simulink model "HSat_orbit"  (R2023a)
settings: Solver=FixedStepAuto  StartTime=0  StopTime=86400*900  MaxStep=3600  RelTol=1e-3  EnableMultiTasking=on
values from neighbouring files (symbols this model uses):
  ext_ENV_G = 6.674e-11    [HSat_op_setup.m]    (also in HSat_op_setup_merged_maria.m)
  ext_ENV_muEarth = 3.986005e14    (= 398600500000000)    [GEO_insertion_setup.m]    (also in HSat_op_setup.m; HSat_op_setup_merged_maria.m; init_orbit_analysis_with_drag_loss.m)
  ext_ENV_Re = 6.37813700*10^6    (= 6378137)    [HSat_op_setup.m]    (also in HSat_op_setup_merged_maria.m)
  ext_EOR_atmosphere_end = 1000e3    (= 1000000)    [HSat_op_setup.m]    (also in HSat_op_setup_merged_maria.m)
  ext_EOR_perigeeraise_end = 600e3    (= 600000)    [HSat_op_setup.m]    (also in HSat_op_setup_merged_maria.m)
  ext_Main_initDate_IC_T = sim_start    [HSat_op_setup.m]    (also in HSat_op_setup_merged_maria.m)
  ext_SC_activecorr_COE_ECI = [1, 1, 1, 0, 0, 0, 0, 0 ]    [HSat_op_setup.m]    (also in HSat_op_setup_merged_maria.m)
  ext_SC_balanced_COE_ECI = [ .500    0.70    1.100 1 1]    [HSat_op_setup.m]    (also in HSat_op_setup_merged_maria.m = [ 0.10 2.10 1.40    1.0000    1.0000]; launch_settings.m)
  ext_SC_cutofferror_COE_ECI = [150e3, .01, 0.1*pi/180, .1*pi/180,.1*pi/180, 0, 0, 0]    [HSat_op_setup.m]    (also in HSat_op_setup_merged_maria.m)
  ext_SC_init_COE_ECI = [a0,ecc0,i0,an0,ap0,tran0,eccan0,ma0]    [HSat_op_setup.m]    (also in HSat_op_setup_merged_maria.m)
  ext_SC_target_COE_ECI = [a1,ecc1,i1,an1,ap1,tran1,eccan1,ma1]    [HSat_op_setup.m]    (also in HSat_op_setup_merged_maria.m)
  ext_SC_target_lambda = 67*pi/180    (= 1.16937059884)    [HSat_op_setup.m]    (also in HSat_op_setup_merged_maria.m)
  sim_SC_init_CoG_EOR_dry = [-0.00448 0.00106 0.46931]    [HSat_op_setup.m]    (also in HSat_op_setup_merged_maria.m)
  sim_SC_init_CoG_propellant = [0 0 0.24758]    [HSat_op_setup.m]    (also in HSat_op_setup_merged_maria.m)
  sim_SC_init_dry_mass = sim_SC_init_wet_mass-sim_SC_init_propellant_mass    (= 727)    [HSat_op_setup.m]    (also in HSat_op_setup_merged_maria.m = 813.7)
  sim_SC_init_wet_mass = 750    [HSat_op_setup.m]    (also in HSat_op_setup_merged_maria.m)
  sim_thrust_force = [ ... (first row only)    [HSat_op_setup.m]    (also in HSat_op_setup_merged_maria.m)
  sim_thrust_massflow = [ ... (first row only)    [HSat_op_setup.m]    (also in HSat_op_setup_merged_maria.m)
  sim_thrust_vector = [ ... (first row only)    [HSat_op_setup.m]    (also in HSat_op_setup_merged_maria.m)
  sim_thruster_position = [ ... (first row only)    [HSat_op_setup.m]    (also in HSat_op_setup_merged_maria.m)
  sim_ts_save = 60    [HSat_op_setup.m]    (also in HSat_op_setup_merged_maria.m)
  third_body_jupiter = 1    [HSat_op_setup.m]    (also in HSat_op_setup_merged_maria.m)
  third_body_moon = 1    [HSat_op_setup.m]    (also in HSat_op_setup_merged_maria.m)
  third_body_sun = 1    [HSat_op_setup.m]    (also in HSat_op_setup_merged_maria.m)
libraries: aerolibutil x26, simulink x12, sharedtransform x7, sharedutil x4, Toolbox x3, matrix_library x1, simulink_extras x1
(part 4 of 5)

== system HSat_orbit/Subsystem1/Subsystem4/Subsystem6/Subsystem2/PPU1+2/VecNormalize1 ==
  In1 : Inport
  Constant : Constant
  Demux : Demux  Outputs=[-1 1]
  Divide : Product  Inputs=*/  OutDataTypeStr=double
  Ground : Ground
  Math Function : Math  Operator=square  SignedPower=on
  Math Function1 : Math  Operator=sqrt  SignedPower=on
  Mux : Mux  Inputs=2
  Mux1 : Mux  Inputs=2
  Product : Product  RndMeth=Zero
  Sum of Elements : Sum  Inputs=+
  Switch : Switch  Criteria=u2 > Threshold  Threshold=eps  SaturateOnIntegerOverflow=off  InputSameDT=off
  Out1 : Outport  VectorParamsAs1DForOutWhenUnconnected=off
  wires:
  Math Function/1 -> Sum of Elements/1
  Demux/1 -> Divide/1
  Constant/1 -> Mux1/2
  Mux1/1 -> Switch/3
  Divide/1 -> Out1/1
  Switch/1 -> Demux/1
  Mux/1 -> Switch/1
  Demux/2 -> Divide/2
  Product/1 -> Mux1/1
  In1/1 -> Product/1, Math Function/1, Mux/1
  Ground/1 -> Product/2
  Sum of Elements/1 -> Math Function1/1
  Math Function1/1 -> Mux/2, Switch/2

== system HSat_orbit/Subsystem1/Subsystem4/Subsystem6/Subsystem2/PPU1+2/VecNormalize2 ==
  In1 : Inport
  Constant : Constant
  Demux : Demux  Outputs=[-1 1]
  Divide : Product  Inputs=*/  OutDataTypeStr=double
  Ground : Ground
  Math Function : Math  Operator=square  SignedPower=on
  Math Function1 : Math  Operator=sqrt  SignedPower=on
  Mux : Mux  Inputs=2
  Mux1 : Mux  Inputs=2
  Product : Product  RndMeth=Zero
  Sum of Elements : Sum  Inputs=+
  Switch : Switch  Criteria=u2 > Threshold  Threshold=eps  SaturateOnIntegerOverflow=off  InputSameDT=off
  Out1 : Outport  VectorParamsAs1DForOutWhenUnconnected=off
  wires:
  Math Function/1 -> Sum of Elements/1
  Demux/1 -> Divide/1
  Constant/1 -> Mux1/2
  Mux1/1 -> Switch/3
  Divide/1 -> Out1/1
  Switch/1 -> Demux/1
  Mux/1 -> Switch/1
  Demux/2 -> Divide/2
  Product/1 -> Mux1/1
  In1/1 -> Product/1, Math Function/1, Mux/1
  Ground/1 -> Product/2
  Sum of Elements/1 -> Math Function1/1
  Math Function1/1 -> Mux/2, Switch/2

== system HSat_orbit/Subsystem1/Subsystem4/Subsystem6/Subsystem2/PPU1+2/VecNormalize3 ==
  In1 : Inport
  Constant : Constant
  Demux : Demux  Outputs=[-1 1]
  Divide : Product  Inputs=*/  OutDataTypeStr=double
  Ground : Ground
  Math Function : Math  Operator=square  SignedPower=on
  Math Function1 : Math  Operator=sqrt  SignedPower=on
  Mux : Mux  Inputs=2
  Mux1 : Mux  Inputs=2
  Product : Product  RndMeth=Zero
  Sum of Elements : Sum  Inputs=+
  Switch : Switch  Criteria=u2 > Threshold  Threshold=eps  SaturateOnIntegerOverflow=off  InputSameDT=off
  Out1 : Outport  VectorParamsAs1DForOutWhenUnconnected=off
  wires:
  Math Function/1 -> Sum of Elements/1
  Demux/1 -> Divide/1
  Constant/1 -> Mux1/2
  Mux1/1 -> Switch/3
  Divide/1 -> Out1/1
  Switch/1 -> Demux/1
  Mux/1 -> Switch/1
  Demux/2 -> Divide/2
  Product/1 -> Mux1/1
  In1/1 -> Product/1, Math Function/1, Mux/1
  Ground/1 -> Product/2
  Sum of Elements/1 -> Math Function1/1
  Math Function1/1 -> Mux/2, Switch/2

== system HSat_orbit/Subsystem1/Subsystem4/Subsystem6/Subsystem2/PPU1+2/VecNormalize4 ==
  In1 : Inport
  Constant : Constant
  Demux : Demux  Outputs=[-1 1]
  Divide : Product  Inputs=*/  OutDataTypeStr=double
  Ground : Ground
  Math Function : Math  Operator=square  SignedPower=on
  Math Function1 : Math  Operator=sqrt  SignedPower=on
  Mux : Mux  Inputs=2
  Mux1 : Mux  Inputs=2
  Product : Product  RndMeth=Zero
  Sum of Elements : Sum  Inputs=+
  Switch : Switch  Criteria=u2 > Threshold  Threshold=eps  SaturateOnIntegerOverflow=off  InputSameDT=off
  Out1 : Outport  VectorParamsAs1DForOutWhenUnconnected=off
  wires:
  Math Function/1 -> Sum of Elements/1
  Demux/1 -> Divide/1
  Constant/1 -> Mux1/2
  Mux1/1 -> Switch/3
  Divide/1 -> Out1/1
  Switch/1 -> Demux/1
  Mux/1 -> Switch/1
  Demux/2 -> Divide/2
  Product/1 -> Mux1/1
  In1/1 -> Product/1, Math Function/1, Mux/1
  Ground/1 -> Product/2
  Sum of Elements/1 -> Math Function1/1
  Math Function1/1 -> Mux/2, Switch/2

== system HSat_orbit/Subsystem1/Subsystem4/Subsystem6/Subsystem2/PPU1+2/VecNormalize5 ==
  In1 : Inport
  Constant : Constant
  Demux : Demux  Outputs=[-1 1]
  Divide : Product  Inputs=*/  OutDataTypeStr=double
  Ground : Ground
  Math Function : Math  Operator=square  SignedPower=on
  Math Function1 : Math  Operator=sqrt  SignedPower=on
  Mux : Mux  Inputs=2
  Mux1 : Mux  Inputs=2
  Product : Product  RndMeth=Zero
  Sum of Elements : Sum  Inputs=+
  Switch : Switch  Criteria=u2 > Threshold  Threshold=eps  SaturateOnIntegerOverflow=off  InputSameDT=off
  Out1 : Outport  VectorParamsAs1DForOutWhenUnconnected=off
  wires:
  Math Function/1 -> Sum of Elements/1
  Demux/1 -> Divide/1
  Constant/1 -> Mux1/2
  Mux1/1 -> Switch/3
  Divide/1 -> Out1/1
  Switch/1 -> Demux/1
  Mux/1 -> Switch/1
  Demux/2 -> Divide/2
  Product/1 -> Mux1/1
  In1/1 -> Product/1, Math Function/1, Mux/1
  Ground/1 -> Product/2
  Sum of Elements/1 -> Math Function1/1
  Math Function1/1 -> Mux/2, Switch/2

== system HSat_orbit/Subsystem1/Subsystem4/Subsystem6/Subsystem2/PPU1+2/VecNormalize6 ==
  In1 : Inport
  Constant : Constant
  Demux : Demux  Outputs=[-1 1]
  Divide : Product  Inputs=*/  OutDataTypeStr=double
  Ground : Ground
  Math Function : Math  Operator=square  SignedPower=on
  Math Function1 : Math  Operator=sqrt  SignedPower=on
  Mux : Mux  Inputs=2
  Mux1 : Mux  Inputs=2
  Product : Product  RndMeth=Zero
  Sum of Elements : Sum  Inputs=+
  Switch : Switch  Criteria=u2 > Threshold  Threshold=eps  SaturateOnIntegerOverflow=off  InputSameDT=off
  Out1 : Outport  VectorParamsAs1DForOutWhenUnconnected=off
  wires:
  Math Function/1 -> Sum of Elements/1
  Demux/1 -> Divide/1
  Constant/1 -> Mux1/2
  Mux1/1 -> Switch/3
  Divide/1 -> Out1/1
  Switch/1 -> Demux/1
  Mux/1 -> Switch/1
  Demux/2 -> Divide/2
  Product/1 -> Mux1/1
  In1/1 -> Product/1, Math Function/1, Mux/1
  Ground/1 -> Product/2
  Sum of Elements/1 -> Math Function1/1
  Math Function1/1 -> Mux/2, Switch/2

== system HSat_orbit/Subsystem1/Subsystem4/Subsystem6/Subsystem2/PPU1+2/VecNormalize7 ==
  In1 : Inport
  Constant : Constant
  Demux : Demux  Outputs=[-1 1]
  Divide : Product  Inputs=*/  OutDataTypeStr=double
  Ground : Ground
  Math Function : Math  Operator=square  SignedPower=on
  Math Function1 : Math  Operator=sqrt  SignedPower=on
  Mux : Mux  Inputs=2
  Mux1 : Mux  Inputs=2
  Product : Product  RndMeth=Zero
  Sum of Elements : Sum  Inputs=+
  Switch : Switch  Criteria=u2 > Threshold  Threshold=eps  SaturateOnIntegerOverflow=off  InputSameDT=off
  Out1 : Outport  VectorParamsAs1DForOutWhenUnconnected=off
  wires:
  Math Function/1 -> Sum of Elements/1
  Demux/1 -> Divide/1
  Constant/1 -> Mux1/2
  Mux1/1 -> Switch/3
  Divide/1 -> Out1/1
  Switch/1 -> Demux/1
  Mux/1 -> Switch/1
  Demux/2 -> Divide/2
  Product/1 -> Mux1/1
  In1/1 -> Product/1, Math Function/1, Mux/1
  Ground/1 -> Product/2
  Sum of Elements/1 -> Math Function1/1
  Math Function1/1 -> Mux/2, Switch/2

== system HSat_orbit/Subsystem1/Subsystem4/Subsystem6/Subsystem2/PPU1+2/VecNormalize8 ==
  In1 : Inport
  Constant : Constant
  Demux : Demux  Outputs=[-1 1]
  Divide : Product  Inputs=*/  OutDataTypeStr=double
  Ground : Ground
  Math Function : Math  Operator=square  SignedPower=on
  Math Function1 : Math  Operator=sqrt  SignedPower=on
  Mux : Mux  Inputs=2
  Mux1 : Mux  Inputs=2
  Product : Product  RndMeth=Zero
  Sum of Elements : Sum  Inputs=+
  Switch : Switch  Criteria=u2 > Threshold  Threshold=eps  SaturateOnIntegerOverflow=off  InputSameDT=off
  Out1 : Outport  VectorParamsAs1DForOutWhenUnconnected=off
  wires:
  Math Function/1 -> Sum of Elements/1
  Demux/1 -> Divide/1
  Constant/1 -> Mux1/2
  Mux1/1 -> Switch/3
  Divide/1 -> Out1/1
  Switch/1 -> Demux/1
  Mux/1 -> Switch/1
  Demux/2 -> Divide/2
  Product/1 -> Mux1/1
  In1/1 -> Product/1, Math Function/1, Mux/1
  Ground/1 -> Product/2
  Sum of Elements/1 -> Math Function1/1
  Math Function1/1 -> Mux/2, Switch/2

== system HSat_orbit/Subsystem1/Subsystem4/Subsystem6/Subsystem2/PPU2/VecNormalize1 ==
  In1 : Inport
  Constant : Constant
  Demux : Demux  Outputs=[-1 1]
  Divide : Product  Inputs=*/  OutDataTypeStr=double
  Ground : Ground
  Math Function : Math  Operator=square  SignedPower=on
  Math Function1 : Math  Operator=sqrt  SignedPower=on
  Mux : Mux  Inputs=2
  Mux1 : Mux  Inputs=2
  Product : Product  RndMeth=Zero
  Sum of Elements : Sum  Inputs=+
  Switch : Switch  Criteria=u2 > Threshold  Threshold=eps  SaturateOnIntegerOverflow=off  InputSameDT=off
  Out1 : Outport  VectorParamsAs1DForOutWhenUnconnected=off
  wires:
  Math Function/1 -> Sum of Elements/1
  Demux/1 -> Divide/1
  Constant/1 -> Mux1/2
  Mux1/1 -> Switch/3
  Divide/1 -> Out1/1
  Switch/1 -> Demux/1
  Mux/1 -> Switch/1
  Demux/2 -> Divide/2
  Product/1 -> Mux1/1
  In1/1 -> Product/1, Math Function/1, Mux/1
  Ground/1 -> Product/2
  Sum of Elements/1 -> Math Function1/1
  Math Function1/1 -> Mux/2, Switch/2

== system HSat_orbit/Subsystem1/Subsystem4/Subsystem6/Subsystem2/PPU2/VecNormalize2 ==
  In1 : Inport
  Constant : Constant
  Demux : Demux  Outputs=[-1 1]
  Divide : Product  Inputs=*/  OutDataTypeStr=double
  Ground : Ground
  Math Function : Math  Operator=square  SignedPower=on
  Math Function1 : Math  Operator=sqrt  SignedPower=on
  Mux : Mux  Inputs=2
  Mux1 : Mux  Inputs=2
  Product : Product  RndMeth=Zero
  Sum of Elements : Sum  Inputs=+
  Switch : Switch  Criteria=u2 > Threshold  Threshold=eps  SaturateOnIntegerOverflow=off  InputSameDT=off
  Out1 : Outport  VectorParamsAs1DForOutWhenUnconnected=off
  wires:
  Math Function/1 -> Sum of Elements/1
  Demux/1 -> Divide/1
  Constant/1 -> Mux1/2
  Mux1/1 -> Switch/3
  Divide/1 -> Out1/1
  Switch/1 -> Demux/1
  Mux/1 -> Switch/1
  Demux/2 -> Divide/2
  Product/1 -> Mux1/1
  In1/1 -> Product/1, Math Function/1, Mux/1
  Ground/1 -> Product/2
  Sum of Elements/1 -> Math Function1/1
  Math Function1/1 -> Mux/2, Switch/2

== system HSat_orbit/Subsystem1/Subsystem4/Subsystem6/Subsystem2/PPU2/VecNormalize3 ==
  In1 : Inport
  Constant : Constant
  Demux : Demux  Outputs=[-1 1]
  Divide : Product  Inputs=*/  OutDataTypeStr=double
  Ground : Ground
  Math Function : Math  Operator=square  SignedPower=on
  Math Function1 : Math  Operator=sqrt  SignedPower=on
  Mux : Mux  Inputs=2
  Mux1 : Mux  Inputs=2
  Product : Product  RndMeth=Zero
  Sum of Elements : Sum  Inputs=+
  Switch : Switch  Criteria=u2 > Threshold  Threshold=eps  SaturateOnIntegerOverflow=off  InputSameDT=off
  Out1 : Outport  VectorParamsAs1DForOutWhenUnconnected=off
  wires:
  Math Function/1 -> Sum of Elements/1
  Demux/1 -> Divide/1
  Constant/1 -> Mux1/2
  Mux1/1 -> Switch/3
  Divide/1 -> Out1/1
  Switch/1 -> Demux/1
  Mux/1 -> Switch/1
  Demux/2 -> Divide/2
  Product/1 -> Mux1/1
  In1/1 -> Product/1, Math Function/1, Mux/1
  Ground/1 -> Product/2
  Sum of Elements/1 -> Math Function1/1
  Math Function1/1 -> Mux/2, Switch/2

== system HSat_orbit/Subsystem1/Subsystem4/Subsystem6/Subsystem2/PPU2/VecNormalize4 ==
  In1 : Inport
  Constant : Constant
  Demux : Demux  Outputs=[-1 1]
  Divide : Product  Inputs=*/  OutDataTypeStr=double
  Ground : Ground
  Math Function : Math  Operator=square  SignedPower=on
  Math Function1 : Math  Operator=sqrt  SignedPower=on
  Mux : Mux  Inputs=2
  Mux1 : Mux  Inputs=2
  Product : Product  RndMeth=Zero
  Sum of Elements : Sum  Inputs=+
  Switch : Switch  Criteria=u2 > Threshold  Threshold=eps  SaturateOnIntegerOverflow=off  InputSameDT=off
  Out1 : Outport  VectorParamsAs1DForOutWhenUnconnected=off
  wires:
  Math Function/1 -> Sum of Elements/1
  Demux/1 -> Divide/1
  Constant/1 -> Mux1/2
  Mux1/1 -> Switch/3
  Divide/1 -> Out1/1
  Switch/1 -> Demux/1
  Mux/1 -> Switch/1
  Demux/2 -> Divide/2
  Product/1 -> Mux1/1
  In1/1 -> Product/1, Math Function/1, Mux/1
  Ground/1 -> Product/2
  Sum of Elements/1 -> Math Function1/1
  Math Function1/1 -> Mux/2, Switch/2

== system HSat_orbit/Subsystem1/Subsystem4/Subsystem6/Subsystem2/PPU2/VecNormalize5 ==
  In1 : Inport
  Constant : Constant
  Demux : Demux  Outputs=[-1 1]
  Divide : Product  Inputs=*/  OutDataTypeStr=double
  Ground : Ground
  Math Function : Math  Operator=square  SignedPower=on
  Math Function1 : Math  Operator=sqrt  SignedPower=on
  Mux : Mux  Inputs=2
  Mux1 : Mux  Inputs=2
  Product : Product  RndMeth=Zero
  Sum of Elements : Sum  Inputs=+
  Switch : Switch  Criteria=u2 > Threshold  Threshold=eps  SaturateOnIntegerOverflow=off  InputSameDT=off
  Out1 : Outport  VectorParamsAs1DForOutWhenUnconnected=off
  wires:
  Math Function/1 -> Sum of Elements/1
  Demux/1 -> Divide/1
  Constant/1 -> Mux1/2
  Mux1/1 -> Switch/3
  Divide/1 -> Out1/1
  Switch/1 -> Demux/1
  Mux/1 -> Switch/1
  Demux/2 -> Divide/2
  Product/1 -> Mux1/1
  In1/1 -> Product/1, Math Function/1, Mux/1
  Ground/1 -> Product/2
  Sum of Elements/1 -> Math Function1/1
  Math Function1/1 -> Mux/2, Switch/2

== system HSat_orbit/Subsystem1/Subsystem4/Subsystem6/Subsystem2/PPU2/VecNormalize6 ==
  In1 : Inport
  Constant : Constant
  Demux : Demux  Outputs=[-1 1]
  Divide : Product  Inputs=*/  OutDataTypeStr=double
  Ground : Ground
  Math Function : Math  Operator=square  SignedPower=on
  Math Function1 : Math  Operator=sqrt  SignedPower=on
  Mux : Mux  Inputs=2
  Mux1 : Mux  Inputs=2
  Product : Product  RndMeth=Zero
  Sum of Elements : Sum  Inputs=+
  Switch : Switch  Criteria=u2 > Threshold  Threshold=eps  SaturateOnIntegerOverflow=off  InputSameDT=off
  Out1 : Outport  VectorParamsAs1DForOutWhenUnconnected=off
  wires:
  Math Function/1 -> Sum of Elements/1
  Demux/1 -> Divide/1
  Constant/1 -> Mux1/2
  Mux1/1 -> Switch/3
  Divide/1 -> Out1/1
  Switch/1 -> Demux/1
  Mux/1 -> Switch/1
  Demux/2 -> Divide/2
  Product/1 -> Mux1/1
  In1/1 -> Product/1, Math Function/1, Mux/1
  Ground/1 -> Product/2
  Sum of Elements/1 -> Math Function1/1
  Math Function1/1 -> Mux/2, Switch/2

== system HSat_orbit/Subsystem1/Subsystem4/Subsystem6/Subsystem2/PPU2/VecNormalize7 ==
  In1 : Inport
  Constant : Constant
  Demux : Demux  Outputs=[-1 1]
  Divide : Product  Inputs=*/  OutDataTypeStr=double
  Ground : Ground
  Math Function : Math  Operator=square  SignedPower=on
  Math Function1 : Math  Operator=sqrt  SignedPower=on
  Mux : Mux  Inputs=2
  Mux1 : Mux  Inputs=2
  Product : Product  RndMeth=Zero
  Sum of Elements : Sum  Inputs=+
  Switch : Switch  Criteria=u2 > Threshold  Threshold=eps  SaturateOnIntegerOverflow=off  InputSameDT=off
  Out1 : Outport  VectorParamsAs1DForOutWhenUnconnected=off
  wires:
  Math Function/1 -> Sum of Elements/1
  Demux/1 -> Divide/1
  Constant/1 -> Mux1/2
  Mux1/1 -> Switch/3
  Divide/1 -> Out1/1
  Switch/1 -> Demux/1
  Mux/1 -> Switch/1
  Demux/2 -> Divide/2
  Product/1 -> Mux1/1
  In1/1 -> Product/1, Math Function/1, Mux/1
  Ground/1 -> Product/2
  Sum of Elements/1 -> Math Function1/1
  Math Function1/1 -> Mux/2, Switch/2

== system HSat_orbit/Subsystem1/Subsystem4/Subsystem6/Subsystem2/PPU2/VecNormalize8 ==
  In1 : Inport
  Constant : Constant
  Demux : Demux  Outputs=[-1 1]
  Divide : Product  Inputs=*/  OutDataTypeStr=double
  Ground : Ground
  Math Function : Math  Operator=square  SignedPower=on
  Math Function1 : Math  Operator=sqrt  SignedPower=on
  Mux : Mux  Inputs=2
  Mux1 : Mux  Inputs=2
  Product : Product  RndMeth=Zero
  Sum of Elements : Sum  Inputs=+
  Switch : Switch  Criteria=u2 > Threshold  Threshold=eps  SaturateOnIntegerOverflow=off  InputSameDT=off
  Out1 : Outport  VectorParamsAs1DForOutWhenUnconnected=off
  wires:
  Math Function/1 -> Sum of Elements/1
  Demux/1 -> Divide/1
  Constant/1 -> Mux1/2
  Mux1/1 -> Switch/3
  Divide/1 -> Out1/1
  Switch/1 -> Demux/1
  Mux/1 -> Switch/1
  Demux/2 -> Divide/2
  Product/1 -> Mux1/1
  In1/1 -> Product/1, Math Function/1, Mux/1
  Ground/1 -> Product/2
  Sum of Elements/1 -> Math Function1/1
  Math Function1/1 -> Mux/2, Switch/2

== system HSat_orbit/Subsystem1/Subsystem4/Subsystem6/Subsystem2/Subsystem1/Subsystem ==
  EORthrustSCB : Inport
  Create 3x3 Matrix : sharedutil/Create 3x3 Matrix  aMode=aMode
      settings: LibrarySourceBlock=aerolibutil/Create 3x3 Matrix
  Demux : Demux  Outputs=3
  Demux1 : Demux  Outputs=3
  Demux2 : Demux  Outputs=3
  Direction Cosine Matrix to Quaternions : sharedtransform/Direction Cosine Matrix  to Quaternions  aMode=0  action=None  tolerance=eps(2)
      settings: LibrarySourceBlock=|
      | aerolibtransform2/Direction Cosine Matrix
      | to Quaternions
  Quaternion Inverse : aerolibutil/Quaternion Inverse
  VecNormalize4 : Subsystem
      mask Display: disp('u/||u||')
  Zeci x Reci : Subsystem  mask(Cross Product){}
      mask help: Calculates the cross product of two 3x1 vectors.
      mask Help:
      | <p>This block calculates the cross product of two 3x1 vectors, ie.</p>
      | 
      | <ul>C(1) = A(2)*B(3) - A(3)*B(2)</ul>
      | <ul>C(2) = A(3)*B(1) - A(1)*B(3)</ul>
      | <ul>C(3) = A(1)*B(2) - A(2)*B(1)</ul>
      | 
      | <p>The block inputs and output contain more than one signal as described below.</p>
      | 
      | <p><H4>Block Vector Input 1 - A</H4>
      | <ul>
      | <li>A(1)</li>
      | <li>A(2)</li>
      | <li>A(3)</li>
      | </ul>
      | </p>
      | 
      | <p><H4>Block Vector Input 2 - B</H4>
      | <ul>
      | <li>B(1)</li>
      | <li>B(2)</li>
      | <li>B(3)</li>
      | </ul>
      | </p>
      | 
      | <p><H4>Block Vector Output - Cross Product (AxB)</H4>
      | <ul>
      | <li>C(1)</li>
      | <li>C(2)</li>
      | <li>C(3)</li>
      | </ul>
      | </p>
      mask Display: disp('Cross\nProduct')
  Zeci x Reci1 : Subsystem  mask(Cross Product){}
      mask help: Calculates the cross product of two 3x1 vectors.
      mask Help:
      | <p>This block calculates the cross product of two 3x1 vectors, ie.</p>
      | 
      | <ul>C(1) = A(2)*B(3) - A(3)*B(2)</ul>
      | <ul>C(2) = A(3)*B(1) - A(1)*B(3)</ul>
      | <ul>C(3) = A(1)*B(2) - A(2)*B(1)</ul>
      | 
      | <p>The block inputs and output contain more than one signal as described below.</p>
      | 
      | <p><H4>Block Vector Input 1 - A</H4>
      | <ul>
      | <li>A(1)</li>
      | <li>A(2)</li>
      | <li>A(3)</li>
      | </ul>
      | </p>
      | 
      | <p><H4>Block Vector Input 2 - B</H4>
      | <ul>
      | <li>B(1)</li>
      | <li>B(2)</li>
      | <li>B(3)</li>
      | </ul>
      | </p>
      | 
      | <p><H4>Block Vector Output - Cross Product (AxB)</H4>
      | <ul>
      | <li>C(1)</li>
      | <li>C(2)</li>
      | <li>C(3)</li>
      | </ul>
      | </p>
      mask Display: disp('Cross\nProduct')
  yscbSCB : Constant  Value=[0 1 0]
  qscbp2scb : Outport
  wires:
  Direction Cosine Matrix to Quaternions/1 -> Quaternion Inverse/1  "qscbp2scb"
  Demux2/3 -> Create 3x3 Matrix/9
  Demux2/1 -> Create 3x3 Matrix/7
  Demux/1 -> Create 3x3 Matrix/1
  Demux1/2 -> Create 3x3 Matrix/5
  EORthrustSCB/1 -> VecNormalize4/1(In1)
  Demux2/2 -> Create 3x3 Matrix/8
  Demux/3 -> Create 3x3 Matrix/3
  Zeci x Reci/1(c(1) c(2) c(3)) -> Zeci x Reci1/2(b(1) b(2) b(3)), Demux/1  "xscbpSCB"
  Demux/2 -> Create 3x3 Matrix/2
  Create 3x3 Matrix/1 -> Direction Cosine Matrix to Quaternions/1
  Zeci x Reci1/1(c(1) c(2) c(3)) -> Demux1/1  "yscbpSCB"
  Demux1/3 -> Create 3x3 Matrix/6
  Demux1/1 -> Create 3x3 Matrix/4
  yscbSCB/1 -> Zeci x Reci/1(a(1) a(2) a(3))
  VecNormalize4/1(Out1) -> Demux2/1, Zeci x Reci1/1(a(1) a(2) a(3)), Zeci x Reci/2(b(1) b(2) b(3))  "zscbpSCB"
  Quaternion Inverse/1 -> qscbp2scb/1

== system HSat_orbit/Subsystem1/Subsystem4/Subsystem6/Subsystem2/Subsystem1/q_scb_calc ==
  torqueECI : Inport
  sunvECI : Inport  Port=2
  Direction Cosine Matrix to Quaternions : sharedtransform/Direction Cosine Matrix  to Quaternions  aMode=0  action=None  tolerance=eps(2)
      settings: LibrarySourceBlock=|
      | aerolibtransform2/Direction Cosine Matrix
      | to Quaternions
  Matrix Concatenate : Concatenate  NumInputs=3  Mode=Multidimensional array
  Reshape1 : Reshape  OutputDimensionality=Row vector (2-D)
  Reshape2 : Reshape  OutputDimensionality=Row vector (2-D)
  Reshape3 : Reshape  OutputDimensionality=Row vector (2-D)
  VecNormalize : Subsystem
      mask Display: disp('u/||u||')
  VecNormalize1 : Subsystem
      mask Display: disp('u/||u||')
  VecNormalize2 : Subsystem
      mask Display: disp('u/||u||')
  VecNormalize3 : Subsystem
      mask Display: disp('u/||u||')
  Yscb x Zscb : Subsystem  mask(Cross Product){}
      mask help: Calculates the cross product of two 3x1 vectors.
      mask Help:
      | <p>This block calculates the cross product of two 3x1 vectors, ie.</p>
      | 
      | <ul>C(1) = A(2)*B(3) - A(3)*B(2)</ul>
      | <ul>C(2) = A(3)*B(1) - A(1)*B(3)</ul>
      | <ul>C(3) = A(1)*B(2) - A(2)*B(1)</ul>
      | 
      | <p>The block inputs and output contain more than one signal as described below.</p>
      | 
      | <p><H4>Block Vector Input 1 - A</H4>
      | <ul>
      | <li>A(1)</li>
      | <li>A(2)</li>
      | <li>A(3)</li>
      | </ul>
      | </p>
      | 
      | <p><H4>Block Vector Input 2 - B</H4>
      | <ul>
      | <li>B(1)</li>
      | <li>B(2)</li>
      | <li>B(3)</li>
      | </ul>
      | </p>
      | 
      | <p><H4>Block Vector Output - Cross Product (AxB)</H4>
      | <ul>
      | <li>C(1)</li>
      | <li>C(2)</li>
      | <li>C(3)</li>
      | </ul>
      | </p>
      mask Display: disp('Cross\nProduct')
  Zeci x Reci : Subsystem  mask(Cross Product){}
      mask help: Calculates the cross product of two 3x1 vectors.
      mask Help:
      | <p>This block calculates the cross product of two 3x1 vectors, ie.</p>
      | 
      | <ul>C(1) = A(2)*B(3) - A(3)*B(2)</ul>
      | <ul>C(2) = A(3)*B(1) - A(1)*B(3)</ul>
      | <ul>C(3) = A(1)*B(2) - A(2)*B(1)</ul>
      | 
      | <p>The block inputs and output contain more than one signal as described below.</p>
      | 
      | <p><H4>Block Vector Input 1 - A</H4>
      | <ul>
      | <li>A(1)</li>
      | <li>A(2)</li>
      | <li>A(3)</li>
      | </ul>
      | </p>
      | 
      | <p><H4>Block Vector Input 2 - B</H4>
      | <ul>
      | <li>B(1)</li>
      | <li>B(2)</li>
      | <li>B(3)</li>
      | </ul>
      | </p>
      | 
      | <p><H4>Block Vector Output - Cross Product (AxB)</H4>
      | <ul>
      | <li>C(1)</li>
      | <li>C(2)</li>
      | <li>C(3)</li>
      | </ul>
      | </p>
      mask Display: disp('Cross\nProduct')
  qECI2scbp : Outport  InitialOutput=0
  wires:
  Zeci x Reci/1(c(1) c(2) c(3)) -> VecNormalize3/1(In1)  "Y"
  VecNormalize1/1(Out1) -> Yscb x Zscb/2(b(1) b(2) b(3)), Reshape3/1, Zeci x Reci/2(b(1) b(2) b(3))  "Zscbp"
  Direction Cosine Matrix to Quaternions/1 -> qECI2scbp/1
  torqueECI/1 -> VecNormalize1/1(In1)
  VecNormalize3/1(Out1) -> Reshape1/1, Yscb x Zscb/1(a(1) a(2) a(3))  "Yscbp"
  Yscb x Zscb/1(c(1) c(2) c(3)) -> VecNormalize/1(In1)
  sunvECI/1 -> VecNormalize2/1(In1)
  Reshape1/1 -> Matrix Concatenate/2
  Reshape3/1 -> Matrix Concatenate/3
  Reshape2/1 -> Matrix Concatenate/1
  VecNormalize/1(Out1) -> Reshape2/1  "Xscbp"
  VecNormalize2/1(Out1) -> Zeci x Reci/1(a(1) a(2) a(3))
  Matrix Concatenate/1 -> Direction Cosine Matrix to Quaternions/1

== system HSat_orbit/Subsystem1/Navigation/Subsystem/Subsystem2/Subsystem7/Subsystem1/Norm4 ==
  In1 : Inport
  Dot Product : DotProduct  OutDataTypeStr=Inherit: Inherit via internal rule
  Sqrt : Sqrt
  Out1 : Outport
  wires:
  In1/1 -> Dot Product/1, Dot Product/2
  Sqrt/1 -> Out1/1
  Dot Product/1 -> Sqrt/1

== system HSat_orbit/Subsystem1/Navigation/Subsystem/Subsystem2/Subsystem7/Subsystem2/Norm3 ==
  In1 : Inport
  Dot Product : DotProduct  OutDataTypeStr=Inherit: Inherit via internal rule
  Sqrt : Sqrt
  Out1 : Outport
  wires:
  In1/1 -> Dot Product/1, Dot Product/2
  Sqrt/1 -> Out1/1
  Dot Product/1 -> Sqrt/1

== system HSat_orbit/Subsystem1/Navigation/Subsystem/Subsystem2/Subsystem7/Subsystem3/Norm5 ==
  In1 : Inport
  Dot Product : DotProduct  OutDataTypeStr=Inherit: Inherit via internal rule
  Sqrt : Sqrt
  Out1 : Outport
  wires:
  In1/1 -> Dot Product/1, Dot Product/2
  Sqrt/1 -> Out1/1
  Dot Product/1 -> Sqrt/1

== system HSat_orbit/Subsystem1/Navigation/Subsystem/Subsystem2/Subsystem7/Subsystem5/Subsystem ==
  nu : Inport
  eabs : Inport  Port=2
  Constant1 : Constant
  Constant2 : Constant  Value=2*pi
  Divide1 : Product  Inputs=**
  Math Function : Math  Operator=square
  Math Function1 : Math  Operator=mod
  Sqrt : Sqrt
  Sum1 : Sum  Inputs=|+-
  Sum3 : Sum  Inputs=|++
  Trigonometric Function1 : Trigonometry  Operator=atan2
  Trigonometric Function2 : Trigonometry  Operator=cos
  Trigonometric Function3 : Trigonometry
  E : Outport
  wires:
  eabs/1 -> Math Function/1, Sum3/1
  nu/1 -> Trigonometric Function3/1, Trigonometric Function2/1
  Trigonometric Function2/1 -> Sum3/2
  Sum3/1 -> Trigonometric Function1/2
  Trigonometric Function1/1 -> Math Function1/1
  Sum1/1 -> Sqrt/1
  Math Function/1 -> Sum1/2
  Constant1/1 -> Sum1/1
  Sqrt/1 -> Divide1/1
  Trigonometric Function3/1 -> Divide1/2
  Divide1/1 -> Trigonometric Function1/1
  Math Function1/1 -> E/1
  Constant2/1 -> Math Function1/2

== system HSat_orbit/Subsystem1/Navigation/Subsystem/Subsystem2/Subsystem7/Subsystem5/Subsystem1 ==
  E : Inport
  eabs : Inport  Port=2
  Constant2 : Constant  Value=2*pi
  Divide1 : Product  Inputs=**
  Math Function1 : Math  Operator=mod
  Sum : Sum  Inputs=|+-
  Trigonometric Function1 : Trigonometry
  M : Outport
  wires:
  Sum/1 -> Math Function1/1  "M"
  eabs/1 -> Divide1/2
  E/1 -> Sum/1, Trigonometric Function1/1
  Divide1/1 -> Sum/2  "e"
  Trigonometric Function1/1 -> Divide1/1
  Constant2/1 -> Math Function1/2
  Math Function1/1 -> M/1

== system HSat_orbit/Subsystem1/Navigation/Subsystem/Subsystem2/Subsystem7/Subsystem5/Subsystem2 ==
  e : Inport
  r : Inport  Port=2
  eabs : Inport  Port=3
  rabs : Inport  Port=4
  Divide8 : Product  Inputs=*/
  Divide9 : Product  Inputs=**
  Dot Product1 : DotProduct  OutDataTypeStr=Inherit: Inherit via internal rule
  Trigonometric Function2 : Trigonometry  Operator=acos
  nu : Outport
  wires:
  eabs/1 -> Divide9/1
  Trigonometric Function2/1 -> nu/1  "nu"
  r/1 -> Dot Product1/2
  rabs/1 -> Divide9/2
  Divide8/1 -> Trigonometric Function2/1
  e/1 -> Dot Product1/1
  Divide9/1 -> Divide8/2  "e"
  Dot Product1/1 -> Divide8/1

== system HSat_orbit/Subsystem1/Navigation/Subsystem/Subsystem2/Subsystem7/Subsystem5/Subsystem3 ==
  E : Inport
  eabs : Inport  Port=2
  Constant : Constant
  Constant1 : Constant
  Divide2 : Product  Inputs=**
  Divide3 : Product  Inputs=*/
  Gain : Gain  Gain=2
  Gain1 : Gain  Gain=.5
  Sqrt : Sqrt
  Sum1 : Sum  Inputs=|++
  Sum2 : Sum  Inputs=|+-
  Trigonometric Function3 : Trigonometry  Operator=atan
  Trigonometric Function4 : Trigonometry  Operator=tan
  nu : Outport
  wires:
  Sqrt/1 -> Divide2/2
  Gain1/1 -> Trigonometric Function4/1
  Constant1/1 -> Sum2/1
  Sum2/1 -> Divide3/2
  eabs/1 -> Sum2/2, Sum1/2
  E/1 -> Gain1/1
  Sum1/1 -> Divide3/1
  Trigonometric Function3/1 -> Gain/1
  Trigonometric Function4/1 -> Divide2/1
  Divide2/1 -> Trigonometric Function3/1
  Constant/1 -> Sum1/1
  Divide3/1 -> Sqrt/1
  Gain/1 -> nu/1  "E"

== system HSat_orbit/Subsystem1/Subsystem4/EORattitude/Subsystem/Subsystem1/Subsystem/VecNormalize4 ==
  In1 : Inport
  Constant : Constant
  Demux : Demux  Outputs=[-1 1]
  Divide : Product  Inputs=*/  OutDataTypeStr=double
  Ground : Ground
  Math Function : Math  Operator=square  SignedPower=on
  Math Function1 : Math  Operator=sqrt  SignedPower=on
  Mux : Mux  Inputs=2
  Mux1 : Mux  Inputs=2
  Product : Product  RndMeth=Zero
  Sum of Elements : Sum  Inputs=+
  Switch : Switch  Criteria=u2 > Threshold  Threshold=eps  SaturateOnIntegerOverflow=off  InputSameDT=off
  Out1 : Outport  VectorParamsAs1DForOutWhenUnconnected=off
  wires:
  Math Function/1 -> Sum of Elements/1
  Demux/1 -> Divide/1
  Constant/1 -> Mux1/2
  Mux1/1 -> Switch/3
  Divide/1 -> Out1/1
  Switch/1 -> Demux/1
  Mux/1 -> Switch/1
  Demux/2 -> Divide/2
  Product/1 -> Mux1/1
  In1/1 -> Product/1, Math Function/1, Mux/1
  Ground/1 -> Product/2
  Sum of Elements/1 -> Math Function1/1
  Math Function1/1 -> Mux/2, Switch/2

== system HSat_orbit/Subsystem1/Subsystem4/EORattitude/Subsystem/Subsystem1/Subsystem/Zeci x Reci ==
  a(1) a(2) a(3) : Inport
  b(1) b(2) b(3) : Inport  Port=2
  Product : Product  InputSameDT=on  SaturateOnIntegerOverflow=on  OutDataTypeStr=Inherit: Same as first input
  Product1 : Product  InputSameDT=on  SaturateOnIntegerOverflow=on  OutDataTypeStr=Inherit: Same as first input
  Selector : Selector  InputPortWidth=3  IndexOptions=Index vector (dialog)  Indices=[2 3 1]  OutputSizes=1
  Selector1 : Selector  InputPortWidth=3  IndexOptions=Index vector (dialog)  Indices=[3 1 2]  OutputSizes=1
  Selector2 : Selector  InputPortWidth=3  IndexOptions=Index vector (dialog)  Indices=[2 3 1]  OutputSizes=1
  Selector3 : Selector  InputPortWidth=3  IndexOptions=Index vector (dialog)  Indices=[3 1 2]  OutputSizes=1
  Sum : Sum  Inputs=+|-  InputSameDT=on  SaturateOnIntegerOverflow=on  OutDataTypeStr=Inherit: Same as first input
  c(1) c(2) c(3) : Outport  InitialOutput=0
  wires:
  Selector3/1 -> Product1/1
  Selector2/1 -> Product1/2
  Product1/1 -> Sum/2
  Selector1/1 -> Product/2
  Product/1 -> Sum/1
  a(1) a(2) a(3)/1 -> Selector3/1, Selector/1
  Selector/1 -> Product/1
  b(1) b(2) b(3)/1 -> Selector2/1, Selector1/1
  Sum/1 -> c(1) c(2) c(3)/1

== system HSat_orbit/Subsystem1/Subsystem4/EORattitude/Subsystem/Subsystem1/Subsystem/Zeci x Reci1 ==
  a(1) a(2) a(3) : Inport
  b(1) b(2) b(3) : Inport  Port=2
  Product : Product  InputSameDT=on  SaturateOnIntegerOverflow=on  OutDataTypeStr=Inherit: Same as first input
  Product1 : Product  InputSameDT=on  SaturateOnIntegerOverflow=on  OutDataTypeStr=Inherit: Same as first input
  Selector : Selector  InputPortWidth=3  IndexOptions=Index vector (dialog)  Indices=[2 3 1]  OutputSizes=1
  Selector1 : Selector  InputPortWidth=3  IndexOptions=Index vector (dialog)  Indices=[3 1 2]  OutputSizes=1
  Selector2 : Selector  InputPortWidth=3  IndexOptions=Index vector (dialog)  Indices=[2 3 1]  OutputSizes=1
  Selector3 : Selector  InputPortWidth=3  IndexOptions=Index vector (dialog)  Indices=[3 1 2]  OutputSizes=1
  Sum : Sum  Inputs=+|-  InputSameDT=on  SaturateOnIntegerOverflow=on  OutDataTypeStr=Inherit: Same as first input
  c(1) c(2) c(3) : Outport  InitialOutput=0
  wires:
  Selector3/1 -> Product1/1
  Selector2/1 -> Product1/2
  Product1/1 -> Sum/2
  Selector1/1 -> Product/2
  Product/1 -> Sum/1
  a(1) a(2) a(3)/1 -> Selector3/1, Selector/1
  Selector/1 -> Product/1
  b(1) b(2) b(3)/1 -> Selector2/1, Selector1/1
  Sum/1 -> c(1) c(2) c(3)/1

== system HSat_orbit/Subsystem1/Subsystem4/EORattitude/Subsystem/Subsystem1/q_scb_calc/VecNormalize ==
  In1 : Inport
  Constant : Constant
  Demux : Demux  Outputs=[-1 1]
  Divide : Product  Inputs=*/  OutDataTypeStr=double
  Ground : Ground
  Math Function : Math  Operator=square  SignedPower=on
  Math Function1 : Math  Operator=sqrt  SignedPower=on
  Mux : Mux  Inputs=2
  Mux1 : Mux  Inputs=2
  Product : Product  RndMeth=Zero
  Sum of Elements : Sum  Inputs=+
  Switch : Switch  Criteria=u2 > Threshold  Threshold=eps  SaturateOnIntegerOverflow=off  InputSameDT=off
  Out1 : Outport  VectorParamsAs1DForOutWhenUnconnected=off
  wires:
  Math Function/1 -> Sum of Elements/1
  Demux/1 -> Divide/1
  Constant/1 -> Mux1/2
  Mux1/1 -> Switch/3
  Divide/1 -> Out1/1
  Switch/1 -> Demux/1
  Mux/1 -> Switch/1
  Demux/2 -> Divide/2
  Product/1 -> Mux1/1
  In1/1 -> Product/1, Math Function/1, Mux/1
  Ground/1 -> Product/2
  Sum of Elements/1 -> Math Function1/1
  Math Function1/1 -> Mux/2, Switch/2

== system HSat_orbit/Subsystem1/Subsystem4/EORattitude/Subsystem/Subsystem1/q_scb_calc/VecNormalize1 ==
  In1 : Inport
  Constant : Constant
  Demux : Demux  Outputs=[-1 1]
  Divide : Product  Inputs=*/  OutDataTypeStr=double
  Ground : Ground
  Math Function : Math  Operator=square  SignedPower=on
  Math Function1 : Math  Operator=sqrt  SignedPower=on
  Mux : Mux  Inputs=2
  Mux1 : Mux  Inputs=2
  Product : Product  RndMeth=Zero
  Sum of Elements : Sum  Inputs=+
  Switch : Switch  Criteria=u2 > Threshold  Threshold=eps  SaturateOnIntegerOverflow=off  InputSameDT=off
  Out1 : Outport  VectorParamsAs1DForOutWhenUnconnected=off
  wires:
  Math Function/1 -> Sum of Elements/1
  Demux/1 -> Divide/1
  Constant/1 -> Mux1/2
  Mux1/1 -> Switch/3
  Divide/1 -> Out1/1
  Switch/1 -> Demux/1
  Mux/1 -> Switch/1
  Demux/2 -> Divide/2
  Product/1 -> Mux1/1
  In1/1 -> Product/1, Math Function/1, Mux/1
  Ground/1 -> Product/2
  Sum of Elements/1 -> Math Function1/1
  Math Function1/1 -> Mux/2, Switch/2

== system HSat_orbit/Subsystem1/Subsystem4/EORattitude/Subsystem/Subsystem1/q_scb_calc/VecNormalize2 ==
  In1 : Inport
  Constant : Constant
  Demux : Demux  Outputs=[-1 1]
  Divide : Product  Inputs=*/  OutDataTypeStr=double
  Ground : Ground
  Math Function : Math  Operator=square  SignedPower=on
  Math Function1 : Math  Operator=sqrt  SignedPower=on
  Mux : Mux  Inputs=2
  Mux1 : Mux  Inputs=2
  Product : Product  RndMeth=Zero
  Sum of Elements : Sum  Inputs=+
  Switch : Switch  Criteria=u2 > Threshold  Threshold=eps  SaturateOnIntegerOverflow=off  InputSameDT=off
  Out1 : Outport  VectorParamsAs1DForOutWhenUnconnected=off
  wires:
  Math Function/1 -> Sum of Elements/1
  Demux/1 -> Divide/1
  Constant/1 -> Mux1/2
  Mux1/1 -> Switch/3
  Divide/1 -> Out1/1
  Switch/1 -> Demux/1
  Mux/1 -> Switch/1
  Demux/2 -> Divide/2
  Product/1 -> Mux1/1
  In1/1 -> Product/1, Math Function/1, Mux/1
  Ground/1 -> Product/2
  Sum of Elements/1 -> Math Function1/1
  Math Function1/1 -> Mux/2, Switch/2

== system HSat_orbit/Subsystem1/Subsystem4/EORattitude/Subsystem/Subsystem1/q_scb_calc/VecNormalize3 ==
  In1 : Inport
  Constant : Constant
  Demux : Demux  Outputs=[-1 1]
  Divide : Product  Inputs=*/  OutDataTypeStr=double
  Ground : Ground
  Math Function : Math  Operator=square  SignedPower=on
  Math Function1 : Math  Operator=sqrt  SignedPower=on
  Mux : Mux  Inputs=2
  Mux1 : Mux  Inputs=2
  Product : Product  RndMeth=Zero
  Sum of Elements : Sum  Inputs=+
  Switch : Switch  Criteria=u2 > Threshold  Threshold=eps  SaturateOnIntegerOverflow=off  InputSameDT=off
  Out1 : Outport  VectorParamsAs1DForOutWhenUnconnected=off
  wires:
  Math Function/1 -> Sum of Elements/1
  Demux/1 -> Divide/1
  Constant/1 -> Mux1/2
  Mux1/1 -> Switch/3
  Divide/1 -> Out1/1
  Switch/1 -> Demux/1
  Mux/1 -> Switch/1
  Demux/2 -> Divide/2
  Product/1 -> Mux1/1
  In1/1 -> Product/1, Math Function/1, Mux/1
  Ground/1 -> Product/2
  Sum of Elements/1 -> Math Function1/1
  Math Function1/1 -> Mux/2, Switch/2

== system HSat_orbit/Subsystem1/Subsystem4/EORattitude/Subsystem/Subsystem1/q_scb_calc/Yscb x Zscb ==
  a(1) a(2) a(3) : Inport
  b(1) b(2) b(3) : Inport  Port=2
  Product : Product  InputSameDT=on  SaturateOnIntegerOverflow=on  OutDataTypeStr=Inherit: Same as first input
  Product1 : Product  InputSameDT=on  SaturateOnIntegerOverflow=on  OutDataTypeStr=Inherit: Same as first input
  Selector : Selector  InputPortWidth=3  IndexOptions=Index vector (dialog)  Indices=[2 3 1]  OutputSizes=1
  Selector1 : Selector  InputPortWidth=3  IndexOptions=Index vector (dialog)  Indices=[3 1 2]  OutputSizes=1
  Selector2 : Selector  InputPortWidth=3  IndexOptions=Index vector (dialog)  Indices=[2 3 1]  OutputSizes=1
  Selector3 : Selector  InputPortWidth=3  IndexOptions=Index vector (dialog)  Indices=[3 1 2]  OutputSizes=1
  Sum : Sum  Inputs=+|-  InputSameDT=on  SaturateOnIntegerOverflow=on  OutDataTypeStr=Inherit: Same as first input
  c(1) c(2) c(3) : Outport  InitialOutput=0
  wires:
  Sum/1 -> c(1) c(2) c(3)/1
  b(1) b(2) b(3)/1 -> Selector1/1, Selector2/1
  Selector/1 -> Product/1
  a(1) a(2) a(3)/1 -> Selector/1, Selector3/1
  Product/1 -> Sum/1
  Selector1/1 -> Product/2
  Product1/1 -> Sum/2
  Selector2/1 -> Product1/2
  Selector3/1 -> Product1/1

== system HSat_orbit/Subsystem1/Subsystem4/EORattitude/Subsystem/Subsystem1/q_scb_calc/Zeci x Reci ==
  a(1) a(2) a(3) : Inport
  b(1) b(2) b(3) : Inport  Port=2
  Product : Product  InputSameDT=on  SaturateOnIntegerOverflow=on  OutDataTypeStr=Inherit: Same as first input
  Product1 : Product  InputSameDT=on  SaturateOnIntegerOverflow=on  OutDataTypeStr=Inherit: Same as first input
  Selector : Selector  InputPortWidth=3  IndexOptions=Index vector (dialog)  Indices=[2 3 1]  OutputSizes=1
  Selector1 : Selector  InputPortWidth=3  IndexOptions=Index vector (dialog)  Indices=[3 1 2]  OutputSizes=1
  Selector2 : Selector  InputPortWidth=3  IndexOptions=Index vector (dialog)  Indices=[2 3 1]  OutputSizes=1
  Selector3 : Selector  InputPortWidth=3  IndexOptions=Index vector (dialog)  Indices=[3 1 2]  OutputSizes=1
  Sum : Sum  Inputs=+|-  InputSameDT=on  SaturateOnIntegerOverflow=on  OutDataTypeStr=Inherit: Same as first input
  c(1) c(2) c(3) : Outport  InitialOutput=0
  wires:
  Selector3/1 -> Product1/1
  Selector2/1 -> Product1/2
  Product1/1 -> Sum/2
  Selector1/1 -> Product/2
  Product/1 -> Sum/1
  a(1) a(2) a(3)/1 -> Selector3/1, Selector/1
  Selector/1 -> Product/1
  b(1) b(2) b(3)/1 -> Selector2/1, Selector1/1
  Sum/1 -> c(1) c(2) c(3)/1

== system HSat_orbit/Subsystem1/Subsystem4/EORattitude/Subsystem/Subsystem3/FlipSatellite/VecNormalize ==
  In1 : Inport
  Constant : Constant
  Demux : Demux  Outputs=[-1 1]
  Divide : Product  Inputs=*/  OutDataTypeStr=double
  Ground : Ground
  Math Function : Math  Operator=square  SignedPower=on
  Math Function1 : Math  Operator=sqrt  SignedPower=on
  Mux : Mux  Inputs=2
  Mux1 : Mux  Inputs=2
  Product : Product  RndMeth=Zero
  Sum of Elements : Sum  Inputs=+
  Switch : Switch  Criteria=u2 > Threshold  Threshold=eps  SaturateOnIntegerOverflow=off  InputSameDT=off
  Out1 : Outport  VectorParamsAs1DForOutWhenUnconnected=off
  wires:
  Math Function/1 -> Sum of Elements/1
  Demux/1 -> Divide/1
  Constant/1 -> Mux1/2
  Mux1/1 -> Switch/3
  Divide/1 -> Out1/1
  Switch/1 -> Demux/1
  Mux/1 -> Switch/1
  Demux/2 -> Divide/2
  Product/1 -> Mux1/1
  In1/1 -> Product/1, Math Function/1, Mux/1
  Ground/1 -> Product/2
  Sum of Elements/1 -> Math Function1/1
  Math Function1/1 -> Mux/2, Switch/2

== system HSat_orbit/Subsystem1/Subsystem4/EORattitude/Subsystem/Subsystem3/FlipSatellite/VecNormalize1 ==
  In1 : Inport
  Constant : Constant
  Demux : Demux  Outputs=[-1 1]
  Divide : Product  Inputs=*/  OutDataTypeStr=double
  Ground : Ground
  Math Function : Math  Operator=square  SignedPower=on
  Math Function1 : Math  Operator=sqrt  SignedPower=on
  Mux : Mux  Inputs=2
  Mux1 : Mux  Inputs=2
  Product : Product  RndMeth=Zero
  Sum of Elements : Sum  Inputs=+
  Switch : Switch  Criteria=u2 > Threshold  Threshold=eps  SaturateOnIntegerOverflow=off  InputSameDT=off
  Out1 : Outport  VectorParamsAs1DForOutWhenUnconnected=off
  wires:
  Math Function/1 -> Sum of Elements/1
  Demux/1 -> Divide/1
  Constant/1 -> Mux1/2
  Mux1/1 -> Switch/3
  Divide/1 -> Out1/1
  Switch/1 -> Demux/1
  Mux/1 -> Switch/1
  Demux/2 -> Divide/2
  Product/1 -> Mux1/1
  In1/1 -> Product/1, Math Function/1, Mux/1
  Ground/1 -> Product/2
  Sum of Elements/1 -> Math Function1/1
  Math Function1/1 -> Mux/2, Switch/2

== system HSat_orbit/Subsystem1/Subsystem4/EORattitude/Subsystem4/Subsystem1/Subsystem/VecNormalize4 ==
  In1 : Inport
  Constant : Constant
  Demux : Demux  Outputs=[-1 1]
  Divide : Product  Inputs=*/  OutDataTypeStr=double
  Ground : Ground
  Math Function : Math  Operator=square  SignedPower=on
  Math Function1 : Math  Operator=sqrt  SignedPower=on
  Mux : Mux  Inputs=2
  Mux1 : Mux  Inputs=2
  Product : Product  RndMeth=Zero
  Sum of Elements : Sum  Inputs=+
  Switch : Switch  Criteria=u2 > Threshold  Threshold=eps  SaturateOnIntegerOverflow=off  InputSameDT=off
  Out1 : Outport  VectorParamsAs1DForOutWhenUnconnected=off
  wires:
  Math Function/1 -> Sum of Elements/1
  Demux/1 -> Divide/1
  Constant/1 -> Mux1/2
  Mux1/1 -> Switch/3
  Divide/1 -> Out1/1
  Switch/1 -> Demux/1
  Mux/1 -> Switch/1
  Demux/2 -> Divide/2
  Product/1 -> Mux1/1
  In1/1 -> Product/1, Math Function/1, Mux/1
  Ground/1 -> Product/2
  Sum of Elements/1 -> Math Function1/1
  Math Function1/1 -> Mux/2, Switch/2

== system HSat_orbit/Subsystem1/Subsystem4/EORattitude/Subsystem4/Subsystem1/Subsystem/Zeci x Reci ==
  a(1) a(2) a(3) : Inport
  b(1) b(2) b(3) : Inport  Port=2
  Product : Product  InputSameDT=on  SaturateOnIntegerOverflow=on  OutDataTypeStr=Inherit: Same as first input
  Product1 : Product  InputSameDT=on  SaturateOnIntegerOverflow=on  OutDataTypeStr=Inherit: Same as first input
  Selector : Selector  InputPortWidth=3  IndexOptions=Index vector (dialog)  Indices=[2 3 1]  OutputSizes=1
  Selector1 : Selector  InputPortWidth=3  IndexOptions=Index vector (dialog)  Indices=[3 1 2]  OutputSizes=1
  Selector2 : Selector  InputPortWidth=3  IndexOptions=Index vector (dialog)  Indices=[2 3 1]  OutputSizes=1
  Selector3 : Selector  InputPortWidth=3  IndexOptions=Index vector (dialog)  Indices=[3 1 2]  OutputSizes=1
  Sum : Sum  Inputs=+|-  InputSameDT=on  SaturateOnIntegerOverflow=on  OutDataTypeStr=Inherit: Same as first input
  c(1) c(2) c(3) : Outport  InitialOutput=0
  wires:
  Selector3/1 -> Product1/1
  Selector2/1 -> Product1/2
  Product1/1 -> Sum/2
  Selector1/1 -> Product/2
  Product/1 -> Sum/1
  a(1) a(2) a(3)/1 -> Selector3/1, Selector/1
  Selector/1 -> Product/1
  b(1) b(2) b(3)/1 -> Selector2/1, Selector1/1
  Sum/1 -> c(1) c(2) c(3)/1

== system HSat_orbit/Subsystem1/Subsystem4/EORattitude/Subsystem4/Subsystem1/Subsystem/Zeci x Reci1 ==
  a(1) a(2) a(3) : Inport
  b(1) b(2) b(3) : Inport  Port=2
  Product : Product  InputSameDT=on  SaturateOnIntegerOverflow=on  OutDataTypeStr=Inherit: Same as first input
  Product1 : Product  InputSameDT=on  SaturateOnIntegerOverflow=on  OutDataTypeStr=Inherit: Same as first input
  Selector : Selector  InputPortWidth=3  IndexOptions=Index vector (dialog)  Indices=[2 3 1]  OutputSizes=1
  Selector1 : Selector  InputPortWidth=3  IndexOptions=Index vector (dialog)  Indices=[3 1 2]  OutputSizes=1
  Selector2 : Selector  InputPortWidth=3  IndexOptions=Index vector (dialog)  Indices=[2 3 1]  OutputSizes=1
  Selector3 : Selector  InputPortWidth=3  IndexOptions=Index vector (dialog)  Indices=[3 1 2]  OutputSizes=1
  Sum : Sum  Inputs=+|-  InputSameDT=on  SaturateOnIntegerOverflow=on  OutDataTypeStr=Inherit: Same as first input
  c(1) c(2) c(3) : Outport  InitialOutput=0
  wires:
  Selector3/1 -> Product1/1
  Selector2/1 -> Product1/2
  Product1/1 -> Sum/2
  Selector1/1 -> Product/2
  Product/1 -> Sum/1
  a(1) a(2) a(3)/1 -> Selector3/1, Selector/1
  Selector/1 -> Product/1
  b(1) b(2) b(3)/1 -> Selector2/1, Selector1/1
  Sum/1 -> c(1) c(2) c(3)/1

== system HSat_orbit/Subsystem1/Subsystem4/EORattitude/Subsystem4/Subsystem1/q_scb_calc/VecNormalize ==
  In1 : Inport
  Constant : Constant
  Demux : Demux  Outputs=[-1 1]
  Divide : Product  Inputs=*/  OutDataTypeStr=double
  Ground : Ground
  Math Function : Math  Operator=square  SignedPower=on
  Math Function1 : Math  Operator=sqrt  SignedPower=on
  Mux : Mux  Inputs=2
  Mux1 : Mux  Inputs=2
  Product : Product  RndMeth=Zero
  Sum of Elements : Sum  Inputs=+
  Switch : Switch  Criteria=u2 > Threshold  Threshold=eps  SaturateOnIntegerOverflow=off  InputSameDT=off
  Out1 : Outport  VectorParamsAs1DForOutWhenUnconnected=off
  wires:
  Math Function/1 -> Sum of Elements/1
  Demux/1 -> Divide/1
  Constant/1 -> Mux1/2
  Mux1/1 -> Switch/3
  Divide/1 -> Out1/1
  Switch/1 -> Demux/1
  Mux/1 -> Switch/1
  Demux/2 -> Divide/2
  Product/1 -> Mux1/1
  In1/1 -> Product/1, Math Function/1, Mux/1
  Ground/1 -> Product/2
  Sum of Elements/1 -> Math Function1/1
  Math Function1/1 -> Mux/2, Switch/2

== system HSat_orbit/Subsystem1/Subsystem4/EORattitude/Subsystem4/Subsystem1/q_scb_calc/VecNormalize1 ==
  In1 : Inport
  Constant : Constant
  Demux : Demux  Outputs=[-1 1]
  Divide : Product  Inputs=*/  OutDataTypeStr=double
  Ground : Ground
  Math Function : Math  Operator=square  SignedPower=on
  Math Function1 : Math  Operator=sqrt  SignedPower=on
  Mux : Mux  Inputs=2
  Mux1 : Mux  Inputs=2
  Product : Product  RndMeth=Zero
  Sum of Elements : Sum  Inputs=+
  Switch : Switch  Criteria=u2 > Threshold  Threshold=eps  SaturateOnIntegerOverflow=off  InputSameDT=off
  Out1 : Outport  VectorParamsAs1DForOutWhenUnconnected=off
  wires:
  Math Function/1 -> Sum of Elements/1
  Demux/1 -> Divide/1
  Constant/1 -> Mux1/2
  Mux1/1 -> Switch/3
  Divide/1 -> Out1/1
  Switch/1 -> Demux/1
  Mux/1 -> Switch/1
  Demux/2 -> Divide/2
  Product/1 -> Mux1/1
  In1/1 -> Product/1, Math Function/1, Mux/1
  Ground/1 -> Product/2
  Sum of Elements/1 -> Math Function1/1
  Math Function1/1 -> Mux/2, Switch/2

== system HSat_orbit/Subsystem1/Subsystem4/EORattitude/Subsystem4/Subsystem1/q_scb_calc/VecNormalize2 ==
  In1 : Inport
  Constant : Constant
  Demux : Demux  Outputs=[-1 1]
  Divide : Product  Inputs=*/  OutDataTypeStr=double
  Ground : Ground
  Math Function : Math  Operator=square  SignedPower=on
  Math Function1 : Math  Operator=sqrt  SignedPower=on
  Mux : Mux  Inputs=2
  Mux1 : Mux  Inputs=2
  Product : Product  RndMeth=Zero
  Sum of Elements : Sum  Inputs=+
  Switch : Switch  Criteria=u2 > Threshold  Threshold=eps  SaturateOnIntegerOverflow=off  InputSameDT=off
  Out1 : Outport  VectorParamsAs1DForOutWhenUnconnected=off
  wires:
  Math Function/1 -> Sum of Elements/1
  Demux/1 -> Divide/1
  Constant/1 -> Mux1/2
  Mux1/1 -> Switch/3
  Divide/1 -> Out1/1
  Switch/1 -> Demux/1
  Mux/1 -> Switch/1
  Demux/2 -> Divide/2
  Product/1 -> Mux1/1
  In1/1 -> Product/1, Math Function/1, Mux/1
  Ground/1 -> Product/2
  Sum of Elements/1 -> Math Function1/1
  Math Function1/1 -> Mux/2, Switch/2

== system HSat_orbit/Subsystem1/Subsystem4/EORattitude/Subsystem4/Subsystem1/q_scb_calc/VecNormalize3 ==
  In1 : Inport
  Constant : Constant
  Demux : Demux  Outputs=[-1 1]
  Divide : Product  Inputs=*/  OutDataTypeStr=double
  Ground : Ground
  Math Function : Math  Operator=square  SignedPower=on
  Math Function1 : Math  Operator=sqrt  SignedPower=on
  Mux : Mux  Inputs=2
  Mux1 : Mux  Inputs=2
  Product : Product  RndMeth=Zero
  Sum of Elements : Sum  Inputs=+
  Switch : Switch  Criteria=u2 > Threshold  Threshold=eps  SaturateOnIntegerOverflow=off  InputSameDT=off
  Out1 : Outport  VectorParamsAs1DForOutWhenUnconnected=off
  wires:
  Math Function/1 -> Sum of Elements/1
  Demux/1 -> Divide/1
  Constant/1 -> Mux1/2
  Mux1/1 -> Switch/3
  Divide/1 -> Out1/1
  Switch/1 -> Demux/1
  Mux/1 -> Switch/1
  Demux/2 -> Divide/2
  Product/1 -> Mux1/1
  In1/1 -> Product/1, Math Function/1, Mux/1
  Ground/1 -> Product/2
  Sum of Elements/1 -> Math Function1/1
  Math Function1/1 -> Mux/2, Switch/2
